simulink library "sph2cart"  (R2018b)
settings: Solver=VariableStepAuto  StartTime=0.0  StopTime=10.0  RelTol=1e-3
settings Model: Creator=BI28030  LastModifiedBy=BI28030

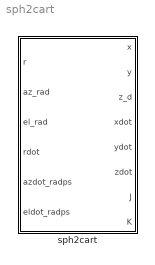
== system sph2cart ==
  sph2cart : MATLAB Function  TreatAsAtomicUnit=on

== matlab function sph2cart/sph2cart ==
  data: x output; r input; az_rad input; el_rad input; y output; z_d output; xdot output; ydot output; zdot output; J output; rdot input; azdot_radps input; eldot_radps input; K output
function [x,y,z_d, xdot,ydot,zdot, J, K] = spherical2cartesian(r,az_rad,el_rad, rdot, azdot_radps, eldot_radps)
%Convert Range, Azimuth, Elevation to North, East, Down coordinates
% Returns the Jacobian J of the 3x3 transformation and the off-diagonal
% Jacobian block K for the 6x6 transformation (so J' = [J zeros(3); K J])

x = r*cos(el_rad)*cos(az_rad);
y = r*cos(el_rad)*sin(az_rad);
z_d = -r*sin(el_rad);

% Jacobian (x,y,z)/(r,az,el)
J = [  x/r  -y   z_d*cos(az_rad); ...
       y/r   x   z_d*sin(az_rad); ...
       z_d/r   0  -r*cos(el_rad) ];
   
% d(x,y,z)/dt = J * d(r,az,el)/dt
xdot = J(1,:)*[rdot; azdot_radps; eldot_radps];
ydot = J(2,:)*[rdot; azdot_radps; eldot_radps];
zdot = J(3,:)*[rdot; azdot_radps; eldot_radps];
   
% position-velocity correlations
Kxdot_r = -(y/r)*azdot_radps + (z_d/r)*cos(az_rad)*eldot_radps;
Kxdot_az = -rdot*(y/r) - x*azdot_radps - z_d*sin(az_rad)*eldot_radps;
Kxdot_el = rdot*(z_d/r)*cos(az_rad) - z_d*sin(az_rad)*azdot_radps - x*eldot_radps;

Kydot_r = (z_d/r)*sin(az_rad)*eldot_radps + (x/r)*azdot_radps;
Kydot_az = rdot*(x/r) + z_d*cos(az_rad)*eldot_radps - y*azdot_radps;
Kydot_el = rdot*(z_d/r)*sin(az_rad) - y*eldot_radps + z_d*cos(az_rad)*azdot_radps;

Kzdot_r = -cos(el_rad)*eldot_radps;
Kzdot_az = 0;
Kzdot_el = -rdot*cos(el_rad) - z_d*eldot_radps;

K = [ Kxdot_r   Kxdot_az   Kxdot_el;
      Kydot_r   Kydot_az   Kydot_el;
      Kzdot_r   Kzdot_az   Kzdot_el   ];
